simulink library "base_lib"  (R2020b)
settings: Solver=VariableStepAuto  StartTime=0.0  StopTime=10.0  RelTol=1e-3
(part 2 of 2)

== matlab function base_lib/F0008_throttle/F0008_throttleFlow2.m ==
  data: p_1 input; W output; p_2 input; T_1 input; T_2 input; alpha input; par parameter
function W = F0008_throttleFlow2(p_1, p_2, T_1, T_2, alpha, par)
% output size
W = zeros(4,1);

% parameters
M_j    = par.M_j;        % [kg/mol] - Molar masses
R_j    = par.R_j;        % [J/kgK]  - Specific gas constants
cp_j   = par.cp_j;       % [J/kgK]  - Specific gas constants

% model parameters
a0 = par.a0;
a1 = par.a1;
a2 = par.a2;

% effective area
A_t = a0 + a1.*alpha + a2 .* alpha.^2;

Pi_lin = par.Pi_lin;

% Pressure & temperature drop
dp = sum(p_1) - sum(p_2);

% Switch variable
dp_tan = dp.*par.tan_par;
y = (tanh(dp_tan) + 1)/2;

% Upstream pressure, temperature & concentration
p_us = y.*p_1 + (1-y).*p_2;
p_ds = y.*p_2 + (1-y).*p_1;
T_us = y.*T_1 + (1-y).*T_2;
T_ds = y.*T_2 + (1-y).*T_1;

% Upstream mole fractions
x_us = p_us ./ sum(p_us);

% Average molar mass
M_avg = sum(x_us .* M_j);

% Mole fraction to mass fraction
w_us = x_us .* M_j ./ M_avg;

% mixture gas constant
R_m  = sum(w_us .* R_j);
cp_m = sum(w_us .* cp_j);
g    = cp_m/(cp_m - R_m);     % [-]      - ratio of specific heats

% pressure ratio
pr = sum(p_ds) ./ sum(p_us);

% primary flow
pr_crit = (2/(1+g)).^( g/(g-1) );
Pi      = max(pr, pr_crit);
Pi      = min(Pi,1);
Phi     = sqrt( 2*g./(g-1) .* ( Pi.^(2/g) - Pi.^((g+1)/g)) );
Phi_lin = sqrt( 2*g./(g-1) .* ( Pi_lin.^(2/g) - Pi_lin.^((g+1)/g)) );
Phi(Pi > Pi_lin) = Phi_lin .* (1-Pi)./(1-Pi_lin);
W_c     = sum(p_us) ./ sqrt(R_m.*T_us) .* A_t .* Phi;
W_c     = W_c .* tanh(dp_tan);

% Distribute mass flow accoring to mass ratios
W   = W_c .* w_us;

== matlab function base_lib/F0009_simpleTractionMotor/F0009_currentDemand.m ==
  data: Tq_em input; Q_gen output; V input; w_em input; I_em output; par parameter
function [Q_gen, I_em] = F0009_currentDemand(Tq_em, V, w_em, par)
% Parameters
e     = par.e;
c1    = par.c1;
c2    = par.c2;
c3    = par.c3;

% Losses
P_0 = c1 + c2 * w_em + c3 * w_em.^2 ;

% Motor power
P_em  = Tq_em .* w_em;
P_el  = e.*P_em + P_0;
I_m   = P_el ./ V;

% Generator power
P_em  = abs(Tq_em) .* w_em;
P_el  = (P_em - P_0)./e;
I_g   = P_el ./ V;

% switching variables
ym = (tanh(Tq_em - pi) + 1)/2;
yg = -(tanh(pi - Tq_em) + 1)/2;

% Current
I_em = ym .* I_m + yg .* I_g;

% Power loss
Q_gen = abs(abs(I_em) .* V - abs(Tq_em .* w_em)); 

end

== matlab function base_lib/F0009_simpleTractionMotor/F0009_torqueLimit.m ==
  data: Tq_req input; Tq_em output; V input; w_em input; par parameter
function Tq_em = F0009_torqueLimit(Tq_req, V, w_em, par)

% Parameters
I_max = par.I_max;
e     = par.e;
c1    = par.c1;
c2    = par.c2;
c3    = par.c3;

% Losses
P_0 = c1 + c2 * w_em + c3 * w_em.^2 ;

% Traction
P_1_trac = I_max .* V;         
P_2_trac = (P_1_trac - P_0)/e;
Tq_trac  = P_2_trac ./ w_em;  % maximum traction torque

% Recuperation
P_1_recup = I_max .* V;
P_2_recup = e.*P_1_recup + P_0;
Tq_recup  = -P_2_recup ./ w_em ;  % minimum recuperation torque

% limit
Tq_em = Tq_req;
Tq_em( Tq_em > Tq_trac)  = Tq_trac;
Tq_em( Tq_em < Tq_recup) = Tq_recup;

end

== matlab function base_lib/F0010_gasFlow/F0010_compressibleRestriction.m ==
  data: p_1 input; W output; p_2 input; T_1 input; T_2 input; open input; par parameter
function W = F0010_compressibleRestriction(p_1, p_2, T_1, T_2, open, par)
% output size
W = zeros(4,1);

% parameters
C_d    = par.C_d;        % [?]      - discharge coefficient
M_j    = par.M_j;        % [kg/mol] - Molar masses
R_j    = par.R_j;        % [J/kgK]  - Specific gas constants
cp_j   = par.cp_j;       % [J/kgK]  - Specific gas constants
D_t    = par.D_t;        % [m]   - Nozzle throat diameter
A_t    = pi*(D_t/2)^2;   % [m2]  - Nozzle throat area

% variable area
A_t    = A_t .* open;

Pi_lin = par.Pi_lin;

% Pressure & temperature drop
dp = sum(p_1) - sum(p_2);

% Switch variable
dp_tan = dp.*par.tan_par;
y = (tanh(dp_tan) + 1)/2;

% Upstream pressure, temperature & concentration
p_us = y.*p_1 + (1-y).*p_2;
p_ds = y.*p_2 + (1-y).*p_1;
T_us = y.*T_1 + (1-y).*T_2;
T_ds = y.*T_2 + (1-y).*T_1;

% Upstream mole fractions
x_us = p_us ./ sum(p_us);

% Average molar mass
M_avg = sum(x_us .* M_j);

% Mole fraction to mass fraction
w_us = x_us .* M_j ./ M_avg;

% mixture gas constant
R_m  = sum(w_us .* R_j);
cp_m = sum(w_us .* cp_j);
g    = cp_m/(cp_m - R_m);     % [-]      - ratio of specific heats

% pressure ratio
pr = sum(p_ds) ./ sum(p_us);

% primary flow
pr_crit = (2/(1+g)).^( g/(g-1) );
Pi      = max(pr, pr_crit);
Pi      = min(Pi,1);
Phi     = sqrt( 2*g./(g-1) .* ( Pi.^(2/g) - Pi.^((g+1)/g)) );
Phi_lin = sqrt( 2*g./(g-1) .* ( Pi_lin.^(2/g) - Pi_lin.^((g+1)/g)) );
Phi(Pi > Pi_lin) = Phi_lin .* (1-Pi)./(1-Pi_lin);
W_c     = sum(p_us) ./ sqrt(R_m.*T_us) .* A_t .* C_d .* Phi;
W_c     = W_c .* tanh(dp_tan);

% Distribute mass flow accoring to mass ratios
W   = W_c .* w_us;

== matlab function base_lib/F0001_panasonicCell/F0001_ocvSOC.m ==
  data: SOC input; U output
function U = F0001_ocvSOC(SOC)
% inputs x [-] - state of charge
% A Generalized SOC-OCV Model for Lithium-Ion
% Batteries and the SOC Estimation for LNMCO Battery
% Zhang et al, Energies
% doi:10.3390/en9110900

% Fit to OCV-data from
% Li-Ion Battery Model Performance for Automotive Drive
% Cycles with Current Pulse and EIS Parameterization
% Kolmeyer et al, 
% 978-1-5090-3953-1/$31.00 ©2017 IEEE

% parameters
a =  2.0966;
b = -0.0055;
c = -0.2433;
d =  2.3054;
m =  3.0965;
n =  0.6010;

% OCV
x = SOC;
U = a + b * (-log(x)).^m + c .* x + d.*exp( n.*(x-1));
end

== matlab function base_lib/F0010_gasFlow/F0010_enthalpyFlow.m ==
  data: W input; H output; T_1 input; T_2 input; par parameter
function H = F0010_enthalpyFlow(W, T_1, T_2, par)
% parameters
cp_j = par.cp_j; % [J/kgK]  - Specific heats

% Upstream & downstream total pressure
% Switch variable
y = (tanh(W*1e4-pi) + 1)/2;

% Upstream temperature
T_us =  y.*T_1 + (1-y).*T_2;

% Enthalpy flow
H = W .* T_us .* cp_j;
end

== matlab function base_lib/F0010_gasFlow/F0010_incompRestr.m ==
  data: p_1 input; W output; T_1 input; p_2 input; T_2 input; par parameter
function W = F0010_incompRestr(p_1, T_1,  p_2, T_2, par)
% output size
W = zeros(4,1);

% parameters
C_d = par.C_d;   % [?]      - Convective flow coefficient
D_t = par.D_t;        % [m]   - Nozzle throat diameter
A_t = pi*(D_t/2)^2;   % [m2]  - Nozzle throat area
M_j = par.M_j; % [kg/mol] - Molar masses
R_j = par.R_j; % [J/kgK]  - Specific gas constants

% Upstream & downstream total pressure
p_1_tot  = sum(p_1);
p_2_tot  = sum(p_2);

% Pressure & temperature drop
dp = p_1_tot - p_2_tot;

dp_tan = dp.*par.tan_par;

% Switch variable
y = (tanh(dp_tan) + 1)/2;

% Upstream pressure, temperature & concentration
p_us = y.*p_1 + (1-y).*p_2;
T_us = y.*T_1 + (1-y).*T_2;

% Upstream total pressure
p_tot = sum(p_us);

% Upstream mole fractions
x_us = p_us ./ p_tot;

% Average molar mass
M_avg = sum(x_us .* M_j);

% Mole fraction to mass fraction
w_us = x_us .* M_j ./ M_avg;

% mixture gas constant
R_m = sum(w_us .* R_j);

% Total mass flow
W_c = C_d .* A_t .* sqrt(p_tot./(R_m.*T_us)).*sqrt(abs(dp));
W_c = tanh(dp_tan) .* W_c;

% linear region
dp_lin  = par.dp_lin;
W_c_lin = C_d .* A_t .* sqrt(p_tot./(R_m.*T_us)) .* abs(dp) ./ sqrt(dp_lin);
W_c(abs(dp) < dp_lin) = tanh(dp_tan) .* W_c_lin;

% Distribute mass flow accoring to mass ratios
W   = W_c .* w_us;
end

== matlab function base_lib/F0010_gasFlow/F0010_linearFlowRestriction.m ==
  data: p_1 input; W output; p_2 input; par parameter
function W = F0010_linearFlowRestriction(p_1,  p_2, par)
% output size
W = zeros(4,1);

% parameters
C_d = par.C_d;   % [?]      - Convective flow coefficient
M_j = par.M_j; % [kg/mol] - Molar masses
R_j = par.R_j; % [J/kgK]  - Specific gas constants

% Upstream & downstream total pressure
p_1_tot  = sum(p_1);
p_2_tot  = sum(p_2);

% Pressure & temperature drop
dp = p_1_tot - p_2_tot;

dp_tan = dp.*par.tan_par;

% Switch variable
y = (tanh(dp_tan) + 1)/2;

% Upstream pressure, temperature & concentration
p_us = y.*p_1 + (1-y).*p_2;

% Upstream total pressure
p_tot = sum(p_us);

% Upstream mole fractions
x_us = p_us ./ p_tot;

% Average molar mass
M_avg = sum(x_us .* M_j);

% Mole fraction to mass fraction
w_us = x_us .* M_j ./ M_avg;

% linear flow
W_c = tanh(dp_tan) .* C_d .* abs(dp) ;

% Distribute mass flow accoring to mass ratios
W   = W_c .* w_us;
end

== matlab function base_lib/F0010_gasFlow/F0010_mixtureMassSpecificHeat.m ==
  data: p input; cp_m output; cv_m output; par parameter
function [cp_m, cv_m] = F0010_mixtureMassSpecificHeat(p, par)
% Parameters
cp_j = par.cp_j; % [J/kgK]  - Specific heats
M_j  = par.M_j;  % [kg/mol] - Molar masses
R_j  = par.R_j;  % [J/kgK]  - Specific gas constant

% Mole fractions
p_tot = sum(p);
x     = p ./ p_tot;

% Average molar mass
M_avg = sum(x .* M_j);

% Mole fraction to mass fraction
w = x .* M_j ./ M_avg;

% Mixture gas constant
R_m = sum(w .* R_j);

% Mixture specific heats
cp_m = sum(w .* cp_j);
cv_m = cp_m - R_m;

end

== matlab function base_lib/F0010_gasFlow/F0010_multicomponentFlow.m ==
  data: p_us input; W_split output; W_tot input; par parameter
function W_split = F0010_multicomponentFlow(p_us, W_tot, par)
% Parameters
cp_j = par.cp_j; % [J/kgK]  - Specific heats
M_j  = par.M_j;  % [kg/mol] - Molar masses
R_j  = par.R_j;  % [J/kgK]  - Specific gas constant

% Mole fractions
p_tot = sum(p_us);
x     = p_us ./ p_tot;

% Average molar mass
M_avg = sum(x .* M_j);

% Mole fraction to mass fraction
w = x .* M_j ./ M_avg;

% outlet species convective mass flow
W_split = W_tot .* w;

end

== matlab function base_lib/F0010_gasFlow/F0010_pressureSupply.m ==
  data: p_tot input; p_out output; x_H2_dry input; x_O2_dry input; RH input; p_sat input; par parameter
function p_out = F0010_pressureSupply(p_tot, x_H2_dry, x_O2_dry, RH, p_sat, par)

% mole fraction of vapor
x_H2O = RH .* p_sat ./ p_tot;

% mole fraction hydrogen
x_H2 = (1-x_H2O).*x_H2_dry;

% mole fraction hydrogen
x_O2 = (1-x_H2O).*x_O2_dry;

% mole fraction nitrogen
x_N2 = 1 - x_H2 - x_O2 - x_H2O;




% partial pressures
p_out = [x_H2; x_O2; x_H2O; x_N2] .* p_tot;

end

== matlab function base_lib/F0010_gasFlow/F0010_pressureToMass.m ==
  data: p input; m output; T input; par parameter
function m = F0010_pressureToMass(p, T, par)
% parameters
Rj     = par.R_j;
V      = par.V;

% mass
m = p .* V ./ (Rj .* T);
end

== matlab function base_lib/F0002_pStack/F0002_pStackVoltage.m ==
  data: I input; V output; T input; Q_gen output; par parameter
function [V, Q_gen] = F0002_pStackVoltage(I, T, par)
% inputs
% i   [A]     - current
% Ta  [K]     - anode inlet temperature
% Tc  [K]     - cathode inlet temperature
% pa  [Pa]    - anode inlet pressure
% pc  [Pa]    - cathode inlet pressure
% TDa [K]     - anode water dewpoint temperature
% TDc [K]     - cathode water dewpoint temperature

% fitting parameters
j_0    = par.j_0;    % [A/cm2]   - exchange current density
alpha  = par.alpha;  % [-]       - reaction transfer coefficient 
ASR    = par.ASR;    % [ohm*cm2] - area-specific resistance
U_0    = par.U_0;    % [V]       - open circuit voltage

% current density
j = I / 300; % [A/cm2];
j = max(j, 0);

% activation voltage
R     = 8.314;
F     = 96485;
V_act = R .* T ./ (alpha.*4.*F) .* log((j+1e-3)./j_0); 

% ohmic losses
V_ohmic = j*ASR;

% total voltage output
V = U_0 - V_act - V_ohmic;

% Heat generation
dh   = 285.8e3;                % [J/mol] - heat of formation (liquid)
% dh     = 241.8e3;                % [J/mol] - heat of formation (vapor)
P_elec = I .* V;              % [W]     - electric power
P_tot  = I ./ (2*F) .* dh;   % [W]     - total power
Q_gen  = P_tot - P_elec;         % [W]     - heat generation

end

== matlab function base_lib/F0011_ellipseCompressor2/F0011_A.m ==
  data: N_corr_n input; A output; par parameter
function A = F0011_A(N_corr_n, par)
% parameters
u1 = N_corr_n;
u2 = par.C_a(1);
u3 = par.C_a(2);
u4 = par.C_a(3);
u5 = par.Delta_h_max;
u6 = par.Wc_max_map;

% output
A = -( u5./u6 ).*( u2.*u1 ./( (1 + u3.*u1.^2).^u4 ));
end

== matlab function base_lib/F0011_ellipseCompressor2/F0011_B.m ==
  data: N_corr_n input; B output; par parameter
function B = F0011_B(N_corr_n, par)
% parameters
u1 = N_corr_n;
u2 = par.C_b(1);
u3 = par.C_b(2);
u4 = par.Delta_h_max;

% output
B = u4 .* ( u2 .* u1.^2 + u3 .* u1^3 );
end

== matlab function base_lib/F0011_ellipseCompressor2/F0011_CUR.m ==
  data: N_corr_n input; CUR output; par parameter
function CUR = F0011_CUR(N_corr_n, par)
% parameters
a1     = par.C_cur(1);
a2     = par.C_cur(2);
a3     = par.C_cur(3);

% Speed ratio
N = N_corr_n;

% output
CUR = a1 + a2.*N.^a3;
end

== matlab function base_lib/F0011_ellipseCompressor2/F0011_K_loss.m ==
  data: W_corr input; K_loss output; N_corr input; par parameter
function K_loss = F0011_K_loss(W_corr, N_corr, par)
% parameters
rho1   = par.rho1;
D      = par.D_2;
C_loss = par.C_loss;

% output
K_loss = 1 + C_loss .* ( rho1.*D.^3 .* pi/60 ) .* (N_corr./W_corr);
end

== matlab function base_lib/F0011_ellipseCompressor2/F0011_PI_ZSL.m ==
  data: N_corr_n input; PI_ZSL output; par parameter
function PI_ZSL = F0011_PI_ZSL(N_corr_n, par)
% parameters
PI_max = par.PI_max_map;
a1     = par.C_PIzs(1);
a2     = par.C_PIzs(2);

% Speed ratio
N = N_corr_n;

% output
PI_ZSL  = 1 + (PI_max - 1) .* ( a1.*N.^a2 );
end

== matlab function base_lib/F0011_ellipseCompressor2/F0011_P_c.m ==
  data: W_c input; P_c output; T_us input; T_ds input; par parameter
function P_c = F0011_P_c(W_c, T_us, T_ds, par)
% parameters
cp  = par.Cp_air;

% compressor work
P_c = cp .* W_c .* (T_ds - T_us);
end

== matlab function base_lib/F0011_ellipseCompressor2/F0011_Pi_ch.m ==
  data: N_corr_n input; Pi_ch output; par parameter
function Pi_ch = F0011_Pi_ch(N_corr_n, par)
% parameters
PI_max = par.PI_max_map;
a1     = par.C_PIch(1);
a2     = par.C_PIch(2);
a3     = par.C_PIch(3);

% Speed ratio
N = N_corr_n;

% output
Pi_ch  = PI_max .* ( a1 + a2.*N.^a3 );
end

== matlab function base_lib/F0011_ellipseCompressor2/F0011_T_ds.m ==
  data: Pi_c input; T_ds output; T_us input; eta_c input; par parameter
function T_ds = F0011_T_ds(Pi_c, T_us, eta_c, par)
% model constants
g = par.gamma_air;

% compressor out temperature (adiabatic)
T_ds = T_us + T_us ./ eta_c .* ( Pi_c.^((g-1)/g)  - 1  );
end

== matlab function base_lib/F0011_ellipseCompressor2/F0011_W_ZSL.m ==
  data: N_corr_n input; W_ZSL output; par parameter
function W_ZSL = F0011_W_ZSL(N_corr_n, par)
% parameters
Wc_max = par.Wc_max_map;
a1     = par.C_Wzs(1);
a2     = par.C_Wzs(2);

% Speed ratio
N = N_corr_n;

% output
W_ZSL = Wc_max .* a1 .* N.^a2;
end

== matlab function base_lib/F0011_ellipseCompressor2/F0011_W_ch_atan.m ==
  data: N_corr_n input; W_ch_atan output; par parameter
function W_ch_atan = F0011_W_ch_atan(N_corr_n, par)
% parameters
Wc_max = par.Wc_max_map;
a1     = par.C_Wch(1);
a2     = par.C_Wch(2);
a3     = par.C_Wch(3);
a4     = par.C_Wch(4);

% Speed ratio
N = N_corr_n;

% output
W_ch_atan = Wc_max .* (a1 + a2 .* atan( a3.*N - a4));
end

== matlab function base_lib/F0011_ellipseCompressor2/F0011_dTq.m ==
  data: Tq_em input; dw_c output; Tq_c input; w_c input; par parameter
function dw_c = F0011_dTq(Tq_em, Tq_c, w_c, par)
% parameters
J_c = par.J_c;
c   = par.c_fric;

% shaft friction
Mf = c .* w_c;

% turbo shaft dynamics
% Model 8.3
dw_c = 1/J_c .* ( Tq_em - Tq_c - Mf);

end

== matlab function base_lib/F0003_pukrushpan2004/F0003_membraneFlow.m ==
  data: lambda_an input; W_an output; lambda_ca input; j input; lambda_m input; T input; W_ca output; par parameter
function [W_an, W_ca] = F0003_membraneFlow(lambda_an, lambda_ca, j, lambda_m, T, par)

% parameters
A   = par.A_fc; % [cm2] - cell area
t_m = par.t_m;  % [cm]  - membrane thickness

% constants
F     = 96485;  % [C/mol]   - Faradays constant
R     = 8.314;  % [J/(molK] - gas constant 
M_H2O = 0.018;  % [kg/mol]  - water molecular mass

rho_mb_dry = 0.002; % [kg/cm^3] - membrane dry density;
M_mb_dry   = 1.1;   % [kg/mol]  - membrane dry equivalent weight 

% electro-osmotic drag coefficient
n_d = 0.0029 .* lambda_m.^2 + 0.05 .* lambda_m;

% membrane diffusivity
D                  = 1e-6;
D(lambda_m >= 2)   = 1e-6 * (1 + 2*(lambda_m-2));
D(lambda_m >= 3)   = 1e-6 * (3 - 1.67*(lambda_m-3));
D(lambda_m >= 4.5) = 1.25e-6;
D_w                = D.*exp(2416*(1/303 - 1/T));

% Water concentrations on each side
c_an = rho_mb_dry ./ M_mb_dry .* lambda_an; % [mol/cm3] - water concentration at anode
c_ca = rho_mb_dry ./ M_mb_dry .* lambda_ca; % [mol/cm3] - water concentration at cathode

% Drag flow
W_drag =   M_H2O .* A .* n_d .* j / F;

% Diffusive flow
W_diff = M_H2O .* A .* D_w .* (c_an - c_ca)/t_m;

% Combined membrane flow
W_m = W_drag + W_diff;

% limits
W_m( lambda_an < 1e-1 & W_m > 0 ) = 0;
W_m( lambda_ca < 1e-1 & W_m < 0 ) = 0;

% output: positive towards cathode
W_an = [0; 0; -W_m; 0];
W_ca = [0; 0;  W_m; 0];
end

== matlab function base_lib/F0011_ellipseCompressor2/F0011_dh_act.m ==
  data: W_c_corr input; dh_act output; K_loss input; B input; A input
function dh_act = F0011_dh_act(W_c_corr, K_loss, B, A)
% inputs
u1 = W_c_corr;
u2 = K_loss;
u3 = B;
u4 = A;

% actual enthalpy change
dh_act = u2 .* ( u3 + u4 .* u1 );
end

== matlab function base_lib/F0011_ellipseCompressor2/F0011_dh_is.m ==
  data: Pi_c input; dh_is output; par parameter
function dh_is = F0011_dh_is(Pi_c, par)
% inputs
u1 = Pi_c;

% parameters
cp_air = par.Cp_air;
T_ref  = par.T_ref;
g      = par.gamma_air;

% isentropic enthalpy change
dh_is = cp_air .* T_ref .* ( u1.^((g - 1)./g) - 1 );
end

== matlab function base_lib/F0011_ellipseCompressor2/F0011_ellipseModel.m ==
  data: Pi_c input; W_corr output; Pi_ch input; PI_ZSL input; CUR input; W_ZSL input; W_ch input; par parameter
function W_corr = F0011_ellipseModel(Pi_c, Pi_ch, PI_ZSL, CUR, W_ZSL, W_ch, par)
% inputs
u1 = min(Pi_c, PI_ZSL);
u2 = Pi_ch;
u3 = PI_ZSL;
u4 = CUR;
u5 = W_ZSL;
u6 = W_ch;

% corrected flow
W = u5 + ...
        (u6-u5) .* ( ...
                        (1 - ( (u1-u2)./(u3-u2) ).^u4).^(1./u4) ...
                    );
                
% surge flow
W_corr_surge = F0011_linearSurgeFlow(W_ZSL, PI_ZSL, Pi_c, par);

% temp flow
W_c = W;

% surge switch
idx       = Pi_c <  PI_ZSL;
W_c(idx)  = W(idx);
W_c(~idx) = W_corr_surge(~idx);

% choke switch
idx       = min(Pi_c,PI_ZSL) <= Pi_ch;
W(idx)    = W_ch(idx);
W(~idx)   = W(~idx);

% output
W_corr = W;
end

== matlab function base_lib/F0011_ellipseCompressor2/F0011_linearSurgeFlow.m ==
  data: W_ZSL input; W_corr_surge output; Pi_ZSL input; Pi_c input; par parameter
function W_corr_surge = F0011_linearSurgeFlow(W_ZSL, Pi_ZSL, Pi_c, par)
% Surge flow
W_corr_surge = W_ZSL - (Pi_c - Pi_ZSL)./par.alpha_kPiW0;

% Saturation
W_corr_surge(W_corr_surge < 1e-4) = 1e-4;
end

== matlab function base_lib/F0011_ellipseCompressor2/F0011_massFlow.m ==
  data: p_1 input; W_c output; p_2 input; T_1 input; w_c input; par parameter
function W_c = F0011_massFlow(p_1, p_2, T_1, w_c, par)
% pressure ratio
Pi_c = p_2 ./ p_1;

% speed correction
[~, N_corr_n] = F0011_speedCorrection(w_c, T_1, par);

% base functions
Pi_ch  = F0011_Pi_ch(N_corr_n, par);
PI_ZSL = F0011_PI_ZSL(N_corr_n, par);
CUR    = F0011_CUR(N_corr_n, par);
W_ZSL  = F0011_W_ZSL(N_corr_n, par);
W_ch   = F0011_W_ch_atan(N_corr_n, par);

% corrected flow
W_corr = F0011_ellipseModel(Pi_c, Pi_ch, PI_ZSL, CUR, W_ZSL, W_ch, par);

% Uncorrect
W_c = W_corr .* (p_1./par.p_ref) ./ sqrt( T_1./par.T_ref);

end

== matlab function base_lib/F0011_ellipseCompressor2/F0011_speedCorrection.m ==
  data: w_c input; N_corr output; T input; N_corr_n output; par parameter
function [N_corr, N_corr_n] = F0011_speedCorrection(w_c, T, par)
% rad/sec -> rpm
N = w_c .* 30/pi;

% speed correction
N_corr = N ./sqrt(T./par.T_ref);

% speed ratio
N_corr_n = N_corr ./ par.Nc_max_map;
end

== matlab function base_lib/F0012_fuelCellThermalCircuit/F0012_anodePlate.m ==
  data: T_m input; dT_an output; T_an input; T_cp input; T_amb input; par parameter
function dT_an = F0012_anodePlate(T_m, T_an, T_cp, T_amb, par)
% parameters
C  = par.C_an;
R4 = par.R4;
R6 = par.R6;
R9 = par.R9;

% output
dT_an = 1./C .*( ...
                    -(1/R4 + 1/R6 + 1/R9).*T_an + ...
                        1/R4 .* T_m  + ...
                        1/R9 .* T_cp + ...
                        1/R6 .* T_amb ...
                );

end

== matlab function base_lib/F0012_fuelCellThermalCircuit/F0012_cathodePlate.m ==
  data: T_m input; dT_ca output; T_ca input; T_cp input; T_amb input; par parameter
function dT_ca = F0012_cathodePlate(T_m, T_ca, T_cp, T_amb, par)
% parameters
C  = par.C_ca;
R5 = par.R5;
R6 = par.R6;
R9 = par.R9;

% output
dT_ca = 1./C .*( ...
                    -(1/R5 + 1/R6 + 1/R9).*T_ca + ...
                        1/R5 .* T_m  + ...
                        1/R9 .* T_cp + ...
                        1/R6 .* T_amb ...
                );
end

== matlab function base_lib/F0012_fuelCellThermalCircuit/F0012_coolantPlate.m ==
  data: T_an input; dT_cp output; T_ca input; T_cp input; Q_cl input; par parameter
function dT_cp = F0012_coolantPlate(T_an, T_ca, T_cp, Q_cl, par)
% parameters
C  = par.C_cp;
R9 = par.R9;

% output
dT_cp = 1./C .*( -2/R9 * T_cp + 1/R9 * T_ca + 1/R9 * T_an - Q_cl);

== matlab function base_lib/F0012_fuelCellThermalCircuit/F0012_coolingPower.m ==
  data: T_cp input; Q_cl output; T_in input; W input; par parameter
function Q_cl = F0012_coolingPower(T_cp, T_in, W, par)
% parameters
hA = par.hA;
cp = par.cp;

% output
Q_cl = 2*hA*W*cp/(hA + 2*W*cp) * (T_cp - T_in);
end

== matlab function base_lib/F0012_fuelCellThermalCircuit/F0012_membraneTemp.m ==
  data: T_an input; T_m output; T_ca input; Q_gen input; par parameter
function T_m = F0012_membraneTemp(T_an, T_ca, Q_gen, par)
% parameters
R4 = par.R4;
R5 = par.R5;

% output
T_m = R5/(R4 + R5) * T_an + R4/(R4 + R5) * T_ca + R4*R5/(R4 + R5) * Q_gen;
end

== matlab function base_lib/F0012_fuelCellThermalCircuit/F0012_outletTemperature.m ==
  data: T_cp input; T_out output; T_in input; W input; par parameter
function T_out = F0012_outletTemperature(T_cp, T_in, W, par)
% parameters
hA = par.hA;
cp = par.cp;

% output
T_out = 2*hA/(hA + 2*W*cp) * T_cp + (2*W*cp - hA)/(hA + 2*W*cp) * T_in;
end

== matlab function base_lib/F0013_simpleEjector/F0013_ejectorModel.m ==
  data: P_p input; W_p output; P_s input; P_b input; T_p input; T_s input; RH_s input; W_s output; phi output; w output; par parameter
function [W_p, W_s, phi, w] = F0013_ejectorModel(P_p, P_s, P_b, T_p, T_s, RH_s, par)

% parameters
C_d    = par.C_d;        % [-]   - Discharge coefficient
D_t    = par.D_t;        % [m]   - Nozzle throat diameter
A_t    = pi*(D_t/2)^2;   % [m2]  - Nozzle throat area
c_0    = par.c_0;
c_1    = par.c_1;
Pi_lin = par.Pi_lin;

% gas properties
M_H2  = 2.016e-3;        % [kg/mol] - hydrogen gas molecular weight
M_H2O = 36.030e-3;       % [kg/mol] - water molecular weight
R_g   = 8.314 / M_H2;    % [J/kg*K] - hydrogen gas constant 
cp    = 14.31e3;         % [J/kg*K] - hydrogen gas specific heat @ 300 K
g     = cp/(cp - R_g);     % [-]      - ratio of specific heats

% pressure ratio
pr = P_b ./ P_p;

% primary flow
pr_crit = (2/(1+g)).^( g/(g-1) );
Pi      = max(pr, pr_crit);
Pi      = min(Pi,1);
Phi     = sqrt( 2*g./(g-1) .* ( Pi.^(2/g) - Pi.^((g+1)/g)) );
Phi_lin = sqrt( 2*g./(g-1) .* ( Pi_lin.^(2/g) - Pi_lin.^((g+1)/g)) );
Phi(Pi > Pi_lin) = Phi_lin .* (1-Pi)./(1-Pi_lin);
W_p     = P_p ./ sqrt(R_g.*T_p) .* A_t .* C_d .* Phi;



% recirculation ratio
t   = ((tanh( (pr - pr_crit)*20 ) ) + 1)/2;
phi = (c_0 + c_1.*pr) .* (1-t); 

% secondary flow
p_sat   = F0003_vaporSaturationPressure(T_s);
x_H2O   = p_sat .* RH_s ./ P_s;
y_H2O   = M_H2O .* x_H2O ./ (M_H2O .* x_H2O + M_H2.*(1 - x_H2O));
W_s     = phi .* W_p ./ (1 - y_H2O);

% entrainment
w = W_s ./ W_p;

== matlab function base_lib/F0003_pukrushpan2004/F0003_outputVoltage.m ==
  data: I input; V output; p_an input; p_ca input; p_sat input; lambda_m input; T input; Q_gen output; par parameter
function [V, Q_gen] = F0003_outputVoltage(I, p_an, p_ca, p_sat, lambda_m, T, par)
% ref: Control-Oriented Modeling and Analysis for Automotive Fuel Cell Systems
% authors: Jay T. Pukrushpan, Huei Peng, Anna G. Stefanopoulou
% J. Dyn. Sys., Meas., Control. Mar 2004
% https://doi.org/10.1115/1.1648308

% specify output sizes
Q_gen = 0;
V     = 0;

% parameters
A = par.A_fc; % [cm2]       - cell area
j = I ./ A;

% partial pressures
p_H2     = p_an(1); % [Pa] - hydrogen partial pressure
% p_H2O_an = p_an(2); % [Pa] - water --
% p_N2_an  = p_an(3); % [Pa] - nitrogen --
p_O2     = p_ca(2); % [Pa] - oxygen --
p_H2O_ca = p_ca(3); % [Pa] - water --
p_N2_ca  = p_ca(4); % [Pa] - nitrogen --

% parameters
c1 = 10;

% constants
R     = 8.314;     % [J/(K mol)] - Gas constant
F     = 96485;     % [C/mol]     - Faradays constant
n     = 2;         % [-]         - moles of electrons transfered per mole hydrogen reacted
E0    = 1.229;     % [V]         - standard potential
P_atm = 1.01325e5; % [Pa]        - atm. pressure
p0    = 1e5;       % [Pa]        - std. pressure
dh    = 285.8e3;   % [J/mol]     - heat of formation (liquid)
% dh    = 241.8e3;   % [J/mol]     - heat of formation (vapor)

% total pressures
% P_an = p_H2 + p_H2O_an + p_N2_an;
P_ca = p_O2 + p_H2O_ca + p_N2_ca;

% reversible voltage
E = E0 - 8.5e-4 .* (T-298.15) + R*T/(n*F) * log(p_H2./p0 .* sqrt(p_O2./p0));

% activation overvoltage
v0 = 0.279 - 8.5e-4 .* (T - 298.15) + 4.3085e-5 .* T .* (log((P_ca/P_atm - p_sat./P_atm)/1.01325) + 1/2 * log(0.1173*(P_ca/P_atm - p_sat./P_atm)/1.01325));
va = (-1.618e-5 * T + 1.618e-2) .* ( p_O2./P_atm./0.1173 + p_sat./P_atm ).^2 + (1.8e-4 * T - 0.166).*(p_O2./ P_atm/0.1173 + p_sat./P_atm) + (-5.8e-4 * T + 0.5736);
V_act = v0 + va.*(1 - exp(-c1.*j));

% ohmic overvoltage
b11     = 0.05139;
b12     = 0.00326;
b2      = 350;
t_m     = 0.01275;
sigma_m = (b11 .* lambda_m - b12) .* exp( b2 .*( 1./303 - 1./T ) );
R_ohm   = t_m ./ sigma_m;
V_ohm   = j .* R_ohm;

% concentration overvoltage
temp         = (p_O2./P_atm./0.1173 + p_sat./P_atm);
c2           = (8.66e-5 .* T - 0.068) .* temp + ( -1.60e-4 * T + 0.54);
c2(temp < 2) = (7.16e-4 .* T - 0.622) .* temp + ( -1.45e-3 * T + 1.68);
c3           = 2;
j_max        = 2.2;
V_con        = j .* (c2 .* j/j_max).^c3;

% Output voltage
V = E  - V_act - V_ohm - V_con;

% Heat generation
P_elec = j.*A .* V;              % [W] - electric power
P_tot  = j .*A ./ (2*F) .* dh;   % [W] - total power
Q_gen  = P_tot - P_elec;         % [W] - heat generation

== matlab function base_lib/F0014_titanXradiator/F0014_condenserPressureDrop.m ==
  data: T input; dp output; p input; W input; par parameter
function dp = F0014_condenserPressureDrop(T, p, W, par)

% parameters
StS  = par.StS;
HtH  = par.HtH;
R    = par.R_air;
c_dp = par.c_dp; 

% Area
A = StS .* HtH;

% Velocity
v = W .* R .* T ./ (p.*A);

% pressure drop
dp = c_dp(1) .* v.^2 + c_dp(2) .* v;

== matlab function base_lib/F0014_titanXradiator/F0014_coreFlowDelay.m ==
  data: W input; t output; par parameter
function t = F0014_coreFlowDelay(W, par)

% parameters
rho = par.rho_clt;
HtH = par.HtH;
StS = par.StS;
CdT = par.CdT;

% approximate core inner flow area
A = 0.15 .* CdT .* StS;

% flow velocity
v = max(W ./ ( rho .* A), 0.01);

% time delay
t = min(HtH ./ v, 20);

== matlab function base_lib/F0014_titanXradiator/F0014_epsCrossFlowUnmixed.m ==
  data: NTU input; e output; C input
function e = F0014_epsCrossFlowUnmixed(NTU, C)
N = NTU;
n = N.^(-0.22);

% tanhyp switch for C approaching zero
y = (tanh(C*1e2 - pi) + 1 )./2;

% Holman, Table 10.3, Cross flow, both fluids unmixed:
e1  = 1 - exp( ( exp( -N.*C.*n ) - 1 )./(C.*n) );

% C = 0
e0 = 1 - exp(-N);

% output
e = y.*e1 + (1-y).*e0;

== matlab function base_lib/F0014_titanXradiator/F0014_fanAffinityLaw.m ==
  data: n1 input; q1 output; q2 input; dp1 output; P1 output; par parameter
function [q1, dp1, P1] = F0014_fanAffinityLaw(n1, q2, par)
% Source:
% https://www.engineeringtoolbox.com/fan-affinity-laws-d_196.html

% parameters
dp2 = par.dp2;
P2  = par.P2;
n2  = par.n2;
d1  = par.d1;
d2  = par.d2;

% Affinity laws
q1  = q2  .* (n1./n2)    .* (d1./d2).^3;
dp1 = dp2 .* (n1./n2).^2 .* (d1./d2).^2;
P1  = P2  .* (n1./n2).^3 .* (d1./d2).^5;

== matlab function base_lib/F0014_titanXradiator/F0014_fanCurve.m ==
  data: q input; dp output; dp0_n input; par parameter
function dp = F0014_fanCurve(q, dp0_n, par)

% parameters
dpr = par.dpr;
dp0 = par.dp0;
q0  = par.q0;

% pressure drop/increase
temp = (q ./ q0).^2;
dp   = max(dpr .* temp, dp0_n - dp0 .* temp);

== matlab function base_lib/F0014_titanXradiator/F0014_heatCapacityRates.m ==
  data: W_air input; C_min output; W_cl input; C_max output; C_air output; C_clt output; par parameter
function [C_min, C_max, C_air, C_clt] = F0014_heatCapacityRates(W_air, W_cl, par)

% parameters
cp_air = par.cp_air;
cp_clt = par.cp_clt;

% heat capacity rates
C_air = W_air.*cp_air;
C_clt = W_cl.*cp_clt;

% max/min rates
C_min = min(C_air, C_clt);
C_max = max(C_air, C_clt);

== matlab function base_lib/F0014_titanXradiator/F0014_intakePressureIncrease.m ==
  data: T input; dp output; p input; v input; par parameter
function dp = F0014_intakePressureIncrease(T, p, v, par)

% parameters
zeta = par.zeta;
R    = par.R_air;

% density
rho = p ./ (R.*T);

% pressure drop
dp = 1/2 .* zeta .* rho .* v.^2;

== matlab function base_lib/F0014_titanXradiator/F0014_radiatorAirPressureDrop.m ==
  data: v input; dp output; par parameter
function dp = F0014_radiatorAirPressureDrop(v, par)
% parameters
CdT   = par.CdT;
c_dp  = par.c_dp_air;
rho   = par.rho_air;

% pressure drop
dp = CdT .* rho .* ( c_dp(1) .* v.^2 + c_dp(2) .* v );

== matlab function base_lib/F0014_titanXradiator/F0014_radiatorCltPressureDrop.m ==
  data: v input; dp output; par parameter
function dp = F0014_radiatorCltPressureDrop(v, par)
% parameters
HtH   = par.HtH;
c_dp  = par.c_dp_clt;
rho   = par.rho_clt;

% pressure drop
dp = HtH .* rho .* ( c_dp(1) .* v.^2 + c_dp(2) .* v );

== matlab function base_lib/F0014_titanXradiator/F0014_restrictionPressureDrop.m ==
  data: T input; dp output; p input; W input; par parameter
function dp = F0014_restrictionPressureDrop(T,p,W,par)

% parameters
zeta = par.zeta;
R    = par.R_air;
A    = par.A;

% density
rho = p ./ (R.*T);

% velocity
v = W ./ (rho.*A);

% pressure drop
dp = 1/2 .* zeta .* rho .* v.^2;

== matlab function base_lib/F0014_titanXradiator/F0014_tankPressureDrop.m ==
  data: v input; dp output; par parameter
function dp = F0014_tankPressureDrop(v, par)
% parameters
zeta = par.zeta;

% pressure drop
dp = 1/2 .* v .* abs(v) .* zeta;

== matlab function base_lib/F0014_titanXradiator/F0014_totalHeatTransferCoefficient.m ==
  data: v_air input; U output; v_clt input; par parameter
function U = F0014_totalHeatTransferCoefficient(v_air, v_clt, par)

% parameters
cU    = par.cU;
cUexp = par.cUexp;

% Heat transfer coefficient
temp = cU(1) + cU(2) .* v_air.^-cUexp(1) + cU(3)*v_clt .^ -cUexp(2);
U    = 1./temp;

== matlab function base_lib/F0015_transmissionControl/F0015_gearSelector.m ==
  data: v input; gear_req output; dV input; gear input
function gear_req   = F0015_gearSelector(v, dV, gear)
%#codegen
% Transmission control unit
switch gear
    case 2 % We are in high gear
        if (v<35)&&(dV<0)
            % we have low speed and deceleration
            gear_req=1;
        else
            gear_req=2;
        end
    case 1 % We are in low gear
        if (v>40)
            gear_req=2;
        else
            gear_req=1;
        end
    otherwise
        disp('Should not be here');
        gear_req=2;
end
            
end

== matlab function base_lib/F0015_transmissionControl/F0015_transmissionControlUnit.m ==
  data: gear_ref input; gear_out output; time input; clutch output
function [gear_out, clutch]  = F0015_transmissionControlUnit(gear_ref,time)
%#codegen
% Transmission control unit
persistent previous_gear incoming_gear last_state
persistent state t_start last_call
t_declutch=0.1;
t_speed_sync=0.2;
t_onclutch=0.1;


% run initialization
if isempty(state)
  % Initial state
  state=0;
  % Need to set varibles (some to dummy) so that codegen gets to know the size of the
  % persistent variables
  previous_gear=2;
  incoming_gear=2;
  t_start=0;
  previous_gear=gear_ref;
  last_call=time;
  last_state=state;
end
  
% Check if Simulink is restarting with smaller step reduction
if time < last_call,
  if state > 0,
    % disp(['Time reversed during gearchange']);
    if time - t_start < t_declutch,
      state=1;
    elseif time - t_start < t_declutch+t_speed_sync,
      state=2;
    elseif time - t_start < t_declutch+t_speed_sync+t_onclutch
      % backing state_machine
      state=3;
    else
      state=0;
    end
  end
end

last_call=time;
last_state=state;

% Run the state machine
switch state,
  case 0, % 'normal'
    if (gear_ref~=previous_gear)
      t_start=time;
      incoming_gear=gear_ref;
      state=1;
    end
    clutch=1;
    gear_out=previous_gear;
  case 1, % 'ramp_down',
    if ((time-t_start)>t_declutch)
      state=2;
      clutch=0;
    else
      clutch=1-(time-t_start)/t_declutch;
    end    
    gear_out=previous_gear;
  case 2, % 'change_gear',
    if (time>(t_start+t_declutch+t_speed_sync))
      state=3; % 'ramp_up';
      clutch=(time-(t_start+t_declutch+t_speed_sync))/t_onclutch;
    else
      clutch=0;
    end
    gear_out=incoming_gear;
  case 3, % 'ramp_up',
    if (time>(t_start+t_declutch+t_speed_sync+t_onclutch))
      state=0; %'normal';
      clutch=1;
    else
      clutch=(time-(t_start+t_declutch+t_speed_sync))/t_onclutch;
    end
    gear_out=incoming_gear;
    previous_gear=incoming_gear;
  otherwise
    error('Unknown state');
end

== matlab function base_lib/F0003_pukrushpan2004/F0003_reactionFlow.m ==
  data: I input; W_an output; W_ca output
function [W_an, W_ca] = F0003_reactionFlow(I)
% constants
F     = 96485; % [C/mol]  - Faradays constant
M_H2  = 0.002; % [kg/mol] - hydrogen molecular weight
M_O2  = 0.032; % [kg/mol] - oxygen   molecular weight
% M_N2  = 0.028; % [kg/mol] - nitrogen molecular weight
M_H2O = 0.018; % [kg/mol] - water    molecular weight

% reaction flows
W_H2_rct  = I * M_H2  /(2*F);
W_O2_rct  = I * M_O2  /(4*F);
W_H2O_rct = I * M_H2O /(2*F);

% output
W_an = [-W_H2_rct;         0;         0; 0];
W_ca = [        0; -W_O2_rct; W_H2O_rct; 0]; 
end

== matlab function base_lib/F0016_speedProfileMPC/F0016_G.m ==
  data: z input; eq output; d input; m input; r_w input; gam input; beta input; dx input
function eq = g(z, d, m, r_w, gam, beta, dx)
% opt. variables
v    = z(1:3:end);
Tq   = z(2:3:end);
u_Tq = z(3:3:end);

% known signals
alpha = d(1:1:end);

% residual vector
eq   = [];

% distance, time, velocity & acceleration
v_i  = ( v(2:end)  + v(1:end-1)) /2;
dv   = v(2:end) - v(1:end-1);
dt   = dx ./ v_i;

% interval driving resistance
alpha_i = ( alpha(2:end) + alpha(1:end-1)  ) /2;
Fg      = m .* 9.82 .* sin(alpha_i);
Fi      = m .* dv./dt;

% tractive force required
Ft      = Fg +  Fi;

% required wheel torque
Tq_w = Ft ./ r_w;

% required motor torque
Tq_req = Tq_w ./ gam;  

% torque balance
Tq_i =( Tq(2:end)  + Tq(1:end-1)) /2;
eq   = [ eq; Tq_req - Tq_i];

% torque dynamics
u_Tq_i = ( u_Tq(2:end) + u_Tq(1:end-1)  ) /2;
eq     = [eq; ((Tq(2:end) - Tq(1:end-1))./dt - beta .* (u_Tq_i - Tq_i))];
end

== matlab function base_lib/F0016_speedProfileMPC/F0016_gradG.m ==
  data: in1 input; dg output; in2 input; m input; r_w input; gam input; beta input; dx input
function dg = grad_g(in1,in2,m,r_w,gam,beta,dx)
%GRAD_G
%    DG = GRAD_G(IN1,IN2,M,R_W,GAM,BETA,DX)

%    This function was generated by the Symbolic Math Toolbox version 8.6.
%    21-Jul-2022 18:47:14

z1 = in1(1,:);
z2 = in1(2,:);
z4 = in1(4,:);
z5 = in1(5,:);
t2 = 1.0./dx;
t3 = 1.0./gam;
t4 = 1.0./r_w;
t5 = -z4;
t6 = -z5;
t7 = beta./2.0;
t8 = z1./2.0;
t9 = z4./2.0;
t10 = t5+z1;
t11 = t6+z2;
t12 = -t7;
t13 = t8+t9;
t14 = (t2.*t11)./2.0;
t15 = (m.*t2.*t10)./2.0;
t17 = t2.*t13;
t16 = -t14;
t18 = m.*t17;
dg = reshape([-t3.*t4.*(t15+t18),t16,-1.0./2.0,t7-t17,0.0,t12,-t3.*t4.*(t15-t18),t16,-1.0./2.0,t7+t17,0.0,t12],[2,6]);

== matlab function base_lib/F0016_speedProfileMPC/F0016_initTrajectories.m ==
  data: v_ref input; v_0 output; alpha input; Tq_0 output; u_Tq_0 output; par parameter
function [v_0, Tq_0, u_Tq_0] = F0016_initTrajectories(v_ref, alpha, par)
% speed linearization
v_0      = repmat(v_ref, 100, 1);

% torque linearization
alpha_i = ( alpha(2:par.N) + alpha(1:par.N-1)  ) /2;
Fg      = par.m .* 9.82 .* sin(alpha_i);
Ft      = Fg;
Tq_w    = Ft ./ par.r_w;
Tq_0    = [Tq_w ./ par.gam; 0];  
u_Tq_0  = Tq_0;
end

== matlab function base_lib/F0016_speedProfileMPC/F0016_qpMatrices.m ==
  data: v_ref input; P output; v input; Tq input; v_0 input; Tq_0 input; u_Tq_0 input; alpha input; c output; A output; b output; G output; h output; par parameter
function [P, c, A, b, G, h] = F0016_qpMatrices(v_ref, v, Tq,  v_0, Tq_0, u_Tq_0, alpha, par)

% variable sizes
nz = 3;
ng = 2;

% parameters
m    = par.m;
r_w  = par.r_w;
gam  = par.gam;
beta = par.beta;
dx   = par.dx;
N    = par.N;


% bounds
v_max   = par.v_max;
v_min   = par.v_min;
Tq_max  = par.Tq_max;
Tq_min  = par.Tq_min;


% previous trajectory
z_0 = [v_0, Tq_0, u_Tq_0]';
z_0 = z_0(:);


% reference
r = [repmat(v_ref, N, 1), Tq_0, u_Tq_0]';
r = r(:);


% linearization trajectory
g_0  = zeros(ng*N-ng, 1);
dg_0 = zeros(length(g_0), length(z_0));


% constraints at t = t0
A_eq_t0       = zeros(2, length(z_0));
A_eq_t0(1,1)  = 1;
A_eq_t0(2,2)  = 1;
b_eq_t0       = [v; Tq];


% constraints at t0 <= t <= tf
for i = 1:N-1
    z_idx = (i*nz+1-nz):(i*nz+nz);
    g_idx = (i*ng+1-ng):(i*ng);
    d_idx = i:(i+1);
    g_0(g_idx)         =     F0016_G( z_0(z_idx), alpha(d_idx), m, r_w, gam, beta, dx );
    dg_0(g_idx, z_idx) = F0016_gradG( z_0(z_idx), alpha(d_idx), m, r_w, gam, beta, dx );
end

% inequality constraints
A_ineq = [];
b_ineq = [];


% equality constraint matrix
A_eq = [A_eq_t0; dg_0];
b_eq = [b_eq_t0; -g_0 + dg_0 * z_0];
A_eq = real(A_eq);
b_eq = real(b_eq);


% cost function
Q     = diag([1 1e-8 1e-8]);
tmp   = repmat({Q}, N, 1);
H     = blkdiag(tmp{:});
H     = (H+H')/2;
f     = - r' * H;


% bounds
LB = repmat([v_min; Tq_min; Tq_min], N, 1);
UB = repmat([v_max; Tq_max; Tq_max], N, 1);
A_bnd = [eye(nz*N); -eye(nz*N)];
b_bnd = [UB; -LB];


% output
P  = H(:);
c  = f;
A  = A_eq(:);
b  = b_eq;
G_ = [A_ineq; A_bnd];
G  = G_(:);
h  = [b_ineq; b_bnd];
end

== matlab function base_lib/F0016_speedProfileMPC/F0016_slopeLookAhead.m ==
  data: full_slope_profile input; slope_lookahead output; x input; par parameter
function slope_lookahead = F0016_slopeLookAhead(full_slope_profile, x, par)

alpha = full_slope_profile;


end

== matlab function base_lib/F0017_channelCooling/F0017_Nusselt.m ==
  data: Re input; Nu output; Pr input; par parameter
function Nu = F0017_Nusselt(Re, Pr, par)

% parameters
d = par.d;
L = par.L;

% Nusselt number relation, J.P Holman eq. 6-9:
Nu = 3.66 + ...
    (0.0668.*(d./L) .* Re .* Pr) ./ ...
    (1 + 0.04 .*( max( (d./L) .* Re .* Pr , 1e-10) ).^(2/3) );

== matlab function base_lib/F0017_channelCooling/F0017_Prandtl.m ==
  data: Pr output; par parameter
function Pr = F0017_Prandtl(par)
% parameters
cp = par.cp_clt;
mu = par.mu_clt;
k  = par.k_clt;

% Prandtl number
Pr = cp .* mu ./ k;

== matlab function base_lib/F0003_pukrushpan2004/F0003_vaporActivity.m ==
  data: p input; a output; P_sat input
function a = F0003_vaporActivity(p, P_sat)
a = p ./ P_sat; % [-] - water vapor activity
end

== matlab function base_lib/F0017_channelCooling/F0017_Reynolds.m ==
  data: v input; Re output; par parameter
function Re = F0017_Reynolds(v, par)
% parameters
rho = par.rho_clt;
mu  = par.mu_clt;
d   = par.d;

% Pipe reynolds number
Re = rho .* v .* d ./ mu;

== matlab function base_lib/F0017_channelCooling/F0017_enthalpyToTemperature.m ==
  data: H input; T output; par parameter
function T = F0017_enthalpyToTemperature(H, par)
    % parameters
    T0 = par.T0_clt;
    H0 = par.H0_clt;
    cp = par.cp_clt;
    
    % temperature
    T = T0 + 1./cp .* (H - H0);

end

== matlab function base_lib/F0017_channelCooling/F0017_heatTransfer.m ==
  data: T_1 input; Q output; T_w input; Nu input; W input; T_2 output; par parameter
function [Q, T_2] = F0017_heatTransfer(T_1, T_w, Nu, W, par)
% Holman example 6-2, Heating of water in Laminar tube flow
% parameters
k  = par.k_clt;
cp = par.cp_clt;
d  = par.d;
L  = par.L;

% heat transfer coefficient
h = k .* Nu ./ d;

% factors
c1 =  W .* cp; 
c2 =  h.*pi.*d.*L;

% outlet temperature
T_2p = (c2 .* T_w + (c1 - c2./2) .* T_1 )./(c1 + c2./2);

% check if temperature reaches wall temperature
if T_1 < T_w
    % cooling
    T_2 = min(T_2p, T_w);
else
    % heating
    T_2 = max(T_2p, T_w);
end
    
% heat transfer
Q = W .* cp .* (T_2 - T_1);

== matlab function base_lib/F0017_channelCooling/F0017_incompressibleRestriction.m ==
  data: W input; dp output; dr input; par parameter
function dp = F0017_incompressibleRestriction(W, dr,  par)

% parameters
C_d = par.C_d;
d   = par.d;
rho = par.rho_clt;

% restriction area
Ar = dr.^2 * pi / 4;

% diameter ratio
beta = dr./d;

% volumetric flow
Q = W ./ rho;

% pressure drop
dp = 1/2 .* rho .* (1 - beta.^4) .* (Q ./ (C_d .* Ar)).^2;

== matlab function base_lib/F0018_ambientProperties/F0018_troposphereModel.m ==
  data: h input; p output; T output; par parameter
function [p,T] = F0018_troposphereModel(h, par)

% parameters
T_0 = par.T_0;
p_0 = par.p_0;

% The nasa troposphere model for pressure.
T = T_0 - 0.00649 .* h;
p = p_0 .* (T./288.078).^5.256;

== matlab function base_lib/F0017_channelCooling/F0017_pressureDrop.m ==
  data: v input; dp output; Re input; par parameter
function dp = F0017_pressureDrop(v, Re,  par)
% parameters
rho = par.rho_clt;
d   = par.d;
L   = par.L;

% Darcy-weisbach friction factor
f = 64 ./ (Re + 0.01);

% pressure drop
dp =  L .* f .* rho./2 .* v.^2 ./ d;

== matlab function base_lib/F0017_channelCooling/F0017_temperatureToEnthalpy.m ==
  data: T input; H output; par parameter
function H = F0017_temperatureToEnthalpy(T, par)
    % parameters
    T0 = par.T0_clt;
    H0 = par.H0_clt;
    cp = par.cp_clt;
    
    % enthalpy
    H = H0 + cp.*(T - T0);

end

== matlab function base_lib/F0010_gasFlow/F0010_vaporSaturationPressure.m ==
  data: T input; p_sat output
function p_sat = F0010_vaporSaturationPressure(T)
% Journal of Physical and Chemical Reference Data 31,
% 387 (2002); https://doi.org/10.1063/1.1461829
c1 =  -7.85951783;
c2 =   1.84408259;
c3 = -11.7866497;
c4 =  22.6807411;
c5 = -15.9618719;
c6 =   1.80122502;

% critical temperature & pressure
Tcrit = 647.096;
pcrit = 22.06e6;

% saturation pressure as function of temperature
p_sat = pcrit*exp(Tcrit./T .* ( ...
    c1*(1-T./Tcrit) + ...
    c2*(1-T./Tcrit).^1.5 + ...
    c3*(1-T./Tcrit).^3 + ...
    c4*(1-T./Tcrit).^3.5 + ...
    c5*(1-T./Tcrit).^4 + ...
    c6*(1-T./Tcrit).^7.5 ));

p_sat = real(p_sat);
end

== matlab function base_lib/F0017_channelCooling/F0017_velocity.m ==
  data: W input; v output; par parameter
function v = F0017_velocity(W, par)

% parameters
rho = par.rho_clt;
d   = par.d;

% area
A = pi .* d.^2 / 4;

% velocity
v = W ./ (rho .* A);

== matlab function base_lib/F0003_pukrushpan2004/F0003_vaporSaturationPressure.m ==
  data: T input; p_sat output
function p_sat = F0003_vaporSaturationPressure(T)
% Journal of Physical and Chemical Reference Data 31,
% 387 (2002); https://doi.org/10.1063/1.1461829
c1 =  -7.85951783;
c2 =   1.84408259;
c3 = -11.7866497;
c4 =  22.6807411;
c5 = -15.9618719;
c6 =   1.80122502;

% critical temperature & pressure
Tcrit = 647.096;
pcrit = 22.06e6;

% saturation pressure as function of temperature
p_sat = pcrit*exp(Tcrit./T .* ( ...
    c1*(1-T./Tcrit) + ...
    c2*(1-T./Tcrit).^1.5 + ...
    c3*(1-T./Tcrit).^3 + ...
    c4*(1-T./Tcrit).^3.5 + ...
    c5*(1-T./Tcrit).^4 + ...
    c6*(1-T./Tcrit).^7.5 ));
end

== matlab function base_lib/F0019_simpleCompressor/F0007_compressorPower.m ==
  data: W_c input; P_c output; T_us input; T_ds input
function P_c = F0007_compressorPower(W_c, T_us, T_ds)

% model constants
g   = 1.4;
R   = 280;
cp  = g*R/(g-1);

% compressor work
% eq. 8.5d
P_c = cp .* W_c .* (T_ds - T_us);

end

== matlab function base_lib/F0019_simpleCompressor/F0007_compressorTemperature.m ==
  data: p_us input; T_ds output; p_ds input; T_us input; eta_c input
function T_ds = F0007_compressorTemperature(p_us, p_ds, T_us, eta_c)

% model constants
g = 1.4;

% pressure ratio
PiC = p_ds./p_us;

% compressor out temperature (adiabatic)
T_ds = T_us + T_us ./ eta_c .* ( PiC.^((g-1)/g)  - 1  );

end

== matlab function base_lib/F0019_simpleCompressor/F0007_multicomponentFlow.m ==
  data: p_us input; W_split output; W_tot input; par parameter
function W_split = F0007_multicomponentFlow(p_us, W_tot, par)
% output size
W = zeros(3,1);

% total pressure
p_tot = sum(p_us);

% partial pressures
p_r  = p_us(1);
p_v  = p_us(2);
p_N2 = p_us(3);

% mole fractions
x_r   = p_r  ./ p_tot;
x_v   = p_v  ./ p_tot;
x_N2  = p_N2 ./ p_tot;

% average mass
M_avg = sum([x_r, x_v, x_N2] .* [par.M_r, par.M_H2O, par.M_N2]);

% mole fraction to mass fraction
w_r   = x_r  .* par.M_r   ./ M_avg;
w_v   = x_v  .* par.M_H2O ./ M_avg;
w_N2  = x_N2 .* par.M_N2  ./ M_avg;

% outlet species convective mass flow
W_split = W_tot .* [w_r; w_v; w_N2];

end
